simulink model "Plant_inversion_perturbed_new_example"  (R2022a)
settings: Solver=ode3  StartTime=-20  StopTime=15  FixedStep=0.001  RelTol=1e-3
settings Model: Creator=Aurelio Piazzi  LastModifiedBy=aurel
settings SolverCC: AlgebraicLoopSolver=TrustRegion
settings DebuggingCC: UnconnectedInputMsg=warning  UnconnectedOutputMsg=warning  UnconnectedLineMsg=warning  SFMachineParentedDataDiag=warning

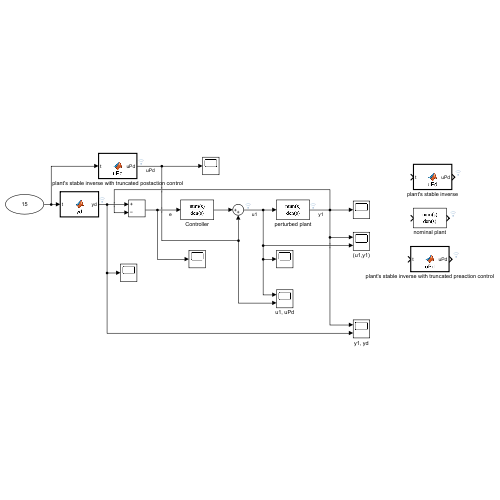
[thumbnail: Simulink's stored preview of the top-level diagram]
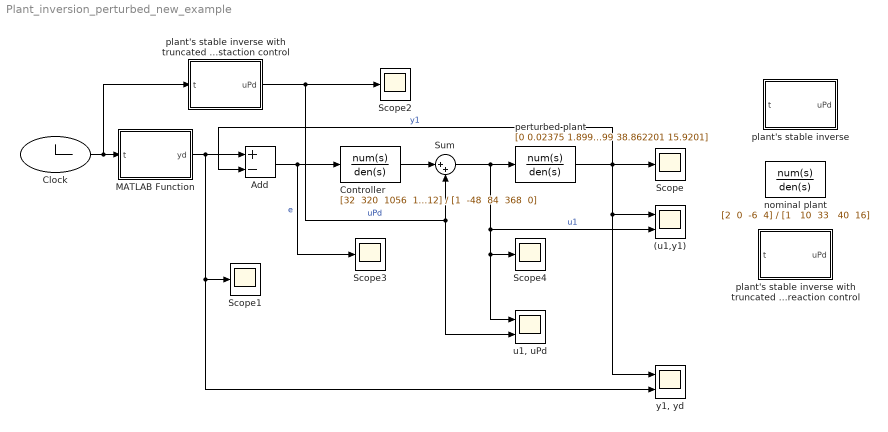
== system Plant_inversion_perturbed_new_example ==
  (u1,y1) : Scope  NumInputPorts=2
  Add : Sum  Inputs=+-
  Clock : Clock
  Controller : TransferFcn  Numerator="[32  320  1056  1280  512]"  Denominator="[1  -48  84  368  0]"
  MATLAB Function : MATLAB Function  TreatAsAtomicUnit=on
  Scope{,1..4} (5 alike) : Scope
  Sum : Sum  Inputs=|++
  nominal plant : TransferFcn  Numerator="[2  0  -6  4]"  Denominator="[1   10  33   40  16]"
  perturbed plant : TransferFcn  Numerator=[0 0.02375 1.89905 -0.141196125 -5.17323188749 3.396649]  Denominator=[0.01 1.097 10.015025 31.8895299 38.862201 15.9201]
  plant's stable inverse : MATLAB Function  TreatAsAtomicUnit=on
  plant's stable inverse with truncated postaction control : MATLAB Function  TreatAsAtomicUnit=on
  plant's stable inverse with truncated preaction control : MATLAB Function  TreatAsAtomicUnit=on
  "u1, uPd" : Scope  NumInputPorts=2
  "y1, yd" : Scope  NumInputPorts=2
  wires:
  MATLAB Function/1(yd) -> "y1, yd"/2, Scope1/1, Add/1
  Add/1 -> Controller/1, Scope3/1  "e"
  perturbed plant/1 -> (u1,y1)/1, "y1, yd"/1, Scope/1, Add/2  "y1"
  Clock/1 -> plant's stable inverse with truncated postaction control/1(t), MATLAB Function/1(t)
  Controller/1 -> Sum/1
  Sum/1 -> (u1,y1)/2, "u1, uPd"/1, Scope4/1, perturbed plant/1  "u1"
  plant's stable inverse with truncated postaction control/1(uPd) -> Scope2/1, "u1, uPd"/2, Sum/2  "uPd"

== matlab function Plant_inversion_perturbed_new_example/MATLAB Function ==
  data: t input; yd output
function yd = yd(t)
 if(t<0)
     yd = 0;
 elseif (t<3)
     yd = (1/3)*t^2-(2/27)*t^3;
 else
     yd = 1;
 end

== matlab function Plant_inversion_perturbed_new_example/plant's stable inverse with truncated preaction control ==
  data: t input; uPd output
function uPd = uPd(t)
% preaction time is equal to 10.17 seconds
if (t<-10.17)
    uPd = 0;
 elseif(t<0)
     uPd = -(20/81)*exp(t)+(8000/81)*exp(-3+t)-(100/27)*exp(t)*t-(500/27)*exp(-3+t)*t;
 elseif (t<3)
     uPd = -2/9-(2/81)*exp(-2*t)+(8000/81)*exp(-3+t)-(500/27)*exp(-3+t)*t-(20/9)*t^2-(8/27)*t^3-(11/3)*t;
 else
     uPd = 4-(2/81)*exp(-2*t)-(1/81)*exp(-2*t+6);
end

== matlab function Plant_inversion_perturbed_new_example/plant's stable inverse ==
  data: t input; uPd output
function uPd = uPd(t)
 if(t<0)
     uPd = -(20/81)*exp(t)+(8000/81)*exp(-3+t)-(100/27)*exp(t)*t-(500/27)*exp(-3+t)*t;
 elseif (t<3)
     uPd = -2/9-(2/81)*exp(-2*t)+(8000/81)*exp(-3+t)-(500/27)*exp(-3+t)*t-(20/9)*t^2-(8/27)*t^3-(11/3)*t;
 else
     uPd = 4-(2/81)*exp(-2*t)-(1/81)*exp(-2*t+6);
 end

== matlab function Plant_inversion_perturbed_new_example/plant's stable inverse with truncated postaction control ==
  data: t input; uPd output
function uPd = uPd(t)
% postaction time is equal to 0.815 seconds
if (t<0)
    uPd = -(20/81)*exp(t)+(8000/81)*exp(-3+t)-(100/27)*exp(t)*t-(500/27)*exp(-3+t)*t;
 elseif (t<3)
    uPd = -2/9-(2/81)*exp(-2*t)+(8000/81)*exp(-3+t)-(500/27)*exp(-3+t)*t-(20/9)*t^2-(8/27)*t^3-(11/3)*t;
 elseif (t < 3 + 0.815)
    uPd = 4-(2/81)*exp(-2*t)-(1/81)*exp(-2*t+6);
else
    uPd = 4;
end
